simulink model "ADP_2LinkRobot_PEFree_ModFree"  (R2018b)
settings: Solver=ode1  StartTime=0.0  StopTime=100  FixedStep=1/1000  RelTol=1e-3  AbsTol=1e-3  EnableMultiTasking=on
PostLoadFcn:
  | f_Simulink_figureplace
InitFcn:
  | ADP_2LinkRobot_PEFree_ModFree_PreSim
values from neighbouring files (symbols this model uses):
  beta = 0.1    [ADP_2LinkRobot_PEFree_ModFree_PreSim.m]
  etaa1 = 5*(projection==0) + 0.1*(projection==1)    [ADP_2LinkRobot_PEFree_ModFree_PreSim.m]
  etaa2 = 0.001*(projection==0)    [ADP_2LinkRobot_PEFree_ModFree_PreSim.m]
  etac1 = 0.5*(projection==0) + 1*(projection==1)    [ADP_2LinkRobot_PEFree_ModFree_PreSim.m]
  etac2 = 10*(projection==0) + 20*(projection==1)    [ADP_2LinkRobot_PEFree_ModFree_PreSim.m]
  F = 9    [ADP_2LinkRobot_PEFree_ModFree_PreSim.m]
  fs = 1000    [ADP_2LinkRobot_PEFree_ModFree_PreSim.m]
  Gamma0 = 100*eye(L)    [ADP_2LinkRobot_PEFree_ModFree_PreSim.m]
  GammaBar = 100000    [ADP_2LinkRobot_PEFree_ModFree_PreSim.m]
  GammaTheta = diag([95 20 170 20])*(projection==0)+     diag([90 40 160 40])*(projection==1)    [ADP_2LinkRobot_PEFree_ModFree_PreSim.m]
  GG = [GG;phi_pc*Gc*(R\Gc')*phi_pc']    [ADP_2LinkRobot_PEFree_ModFree_PreSim.m]
  k = 10    [ADP_2LinkRobot_PEFree_ModFree_PreSim.m]
  kTheta = 1.1*(projection==0) + 1.1*(projection==1)    [ADP_2LinkRobot_PEFree_ModFree_PreSim.m]
  learning = 1    [ADP_2LinkRobot_PEFree_ModFree_PreSim.m]
  M = 20    [ADP_2LinkRobot_PEFree_ModFree_PreSim.m]
  model = 0    [ADP_2LinkRobot_PEFree_ModFree_PreSim.m]
  N = length(Xc)^4    [ADP_2LinkRobot_PEFree_ModFree_PreSim.m]
  pecutoff = 0.4    [ADP_2LinkRobot_PEFree_ModFree_PreSim.m]
  PHIPF1 = zeros(L,N)    [ADP_2LinkRobot_PEFree_ModFree_PreSim.m]
  PHIPY = [PHIPY;phi_pc*Yc]    [ADP_2LinkRobot_PEFree_ModFree_PreSim.m]
  projection = 1    [ADP_2LinkRobot_PEFree_ModFree_PreSim.m]
  Q = [10 0 0 0; 0 10 0 0; 0 0 1 0; 0 0 0 1]    [ADP_2LinkRobot_PEFree_ModFree_PreSim.m]
  R = 1    [ADP_2LinkRobot_PEFree_ModFree_PreSim.m]
  theta0 = 1*[1; 1; 1; 1]    [ADP_2LinkRobot_PEFree_ModFree_PreSim.m]
  typ = 1    [ADP_2LinkRobot_PEFree_ModFree_PreSim.m]
  v = 0.005    [ADP_2LinkRobot_PEFree_ModFree_PreSim.m]
  WaH0 = 1*WcH0    [ADP_2LinkRobot_PEFree_ModFree_PreSim.m]
  WcH0 = [24.6297684659567,1.18840698913485,2.23807515028947,2.63543366699068,1.16589636116696,0.925620360472737,44.2298481912473,11.2724861339746,3.80631458802382,0.112951648575195]    [ADP_2LinkRobot_PEFree_ModFree_PreSim.m]
  x0 = [1;1;0;0]    [ADP_2LinkRobot_PEFree_ModFree_PreSim.m]
  XQX = zeros(N,1)    [ADP_2LinkRobot_PEFree_ModFree_PreSim.m]
undefined symbols (not defined in the file or in its folder): g
settings Model: Creator=rkamalapurkar  LastModifiedBy=rushik
settings SolverCC: AutoScaleAbsTol=off
settings DataIOCC: LimitDataPoints=on  SaveFormat=Array  SignalLoggingSaveFormat=ModelDataLogs
settings OptimizationCC: ExpressionDepthLimit=2147483647  LifeSpan=inf
settings DebuggingCC: UnderspecifiedInitializationDetection=Classic  MergeDetectMultiDrivingBlocksExec=none  SolverPrmCheckMsg=warning  FcnCallInpInsideContextMsg=warning  StateNameClashWarn=warning  SFUnexpectedBacktrackingDiag=warning  SFNoUnconditionalDefaultTransitionDiag=warning  SFExecutionAtInitializationDiag=none
settings HardwareCC: ProdBitPerPointer=32  ProdBitPerSizeT=32  ProdBitPerPtrDiffT=32  ProdLargestAtomicFloat=None  ProdIntDivRoundTo=Undefined  ProdEndianess=Unspecified  ProdWordSize=32  ProdHWDeviceType=32-bit Generic
settings ModelReferenceCC: PropagateSignalLabelsOutOfModel=off
settings SFSimCC: SimUseLocalCustomCode=off
settings RTWCC: RTWUseLocalCustomCode=off
settings CodeAppCC: StateflowObjectComments=on
settings GRTTargetCC: TargetLangStandard=C89/C90 (ANSI)  GeneratePreprocessorConditionals=Disable all  CombineOutputUpdateFcns=off  GRTInterface=on
settings ConfigComp: CovMetricSettings=dw  CovHtmlReporting=on  CovSaveCumulativeToWorkspaceVar=on  CovSaveSingleToWorkspaceVar=on  CovExternalEMLEnable=off  CovSFcnEnable=off

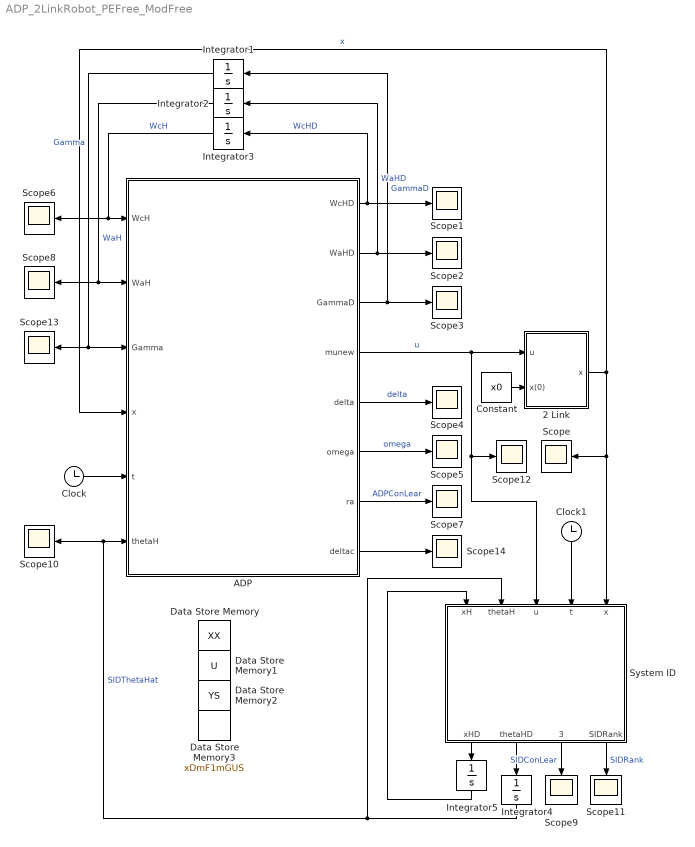
== system ADP_2LinkRobot_PEFree_ModFree ==
  2 Link : Subsystem
  ADP : MATLAB Function  TreatAsAtomicUnit=on
  Clock : Clock
  Clock1 : Clock
  Constant : Constant  Value=x0
  Data Store Memory : DataStoreMemory  DataStoreName=XX  InitialValue=zeros(4,F)  ShowAdditionalParam=off  OutDataTypeStr=double
  Data Store Memory1 : DataStoreMemory  DataStoreName=U  InitialValue=zeros(2,(F+1)/2)  ShowAdditionalParam=off  OutDataTypeStr=double
  Data Store Memory2 : DataStoreMemory  DataStoreName=YS  InitialValue=zeros(4,4*M)  ShowAdditionalParam=off  OutDataTypeStr=double
  Data Store Memory3 : DataStoreMemory  DataStoreName=xDmF1mGUS  InitialValue=zeros(4,M)  ShowAdditionalParam=off  OutDataTypeStr=double
  Integrator1 : Integrator  InitialCondition=Gamma0
  Integrator2 : Integrator  InitialCondition=WaH0
  Integrator3 : Integrator  InitialCondition=WcH0
  Integrator4 : Integrator  InitialCondition=theta0
  Integrator5 : Integrator  InitialCondition=[0;0;0;0]
  Scope{,1..14} (15 alike) : Scope
  System ID : MATLAB Function  TreatAsAtomicUnit=on
  wires:
  ADP/3(GammaD) -> Integrator1/1, Scope3/1  "GammaD"
  ADP/1(WcHD) -> Integrator3/1, Scope1/1  "WcHD"
  Integrator3/1 -> Scope6/1, ADP/1(WcH)  "WcH"
  ADP/2(WaHD) -> Integrator2/1, Scope2/1  "WaHD"
  Integrator2/1 -> ADP/2(WaH), Scope8/1  "WaH"
  ADP/5(delta) -> Scope4/1  "delta"
  ADP/6(omega) -> Scope5/1  "omega"
  Integrator1/1 -> Scope13/1, ADP/3(Gamma)  "Gamma"
  Clock/1 -> ADP/5(t)
  ADP/4(munew) -> System ID/3(u), Scope12/1, 2 Link/1(u)  "u"
  ADP/7(ra) -> Scope7/1  "ADPConLear"
  Integrator4/1 -> System ID/2(thetaH), Scope10/1, ADP/6(thetaH)  "SIDThetaHat"
  2 Link/1(x) -> ADP/4(x), System ID/5(x), Scope/1  "x"
  Constant/1 -> 2 Link/2(x(0))
  System ID/1(xHD) -> Integrator5/1
  Integrator5/1 -> System ID/1(xH)
  System ID/4(SIDRank) -> Scope11/1  "SIDRank"
  System ID/3(SIDConLear) -> Scope9/1  "SIDConLear"
  System ID/2(thetaHD) -> Integrator4/1
  Clock1/1 -> System ID/4(t)
  ADP/8(deltac) -> Scope14/1

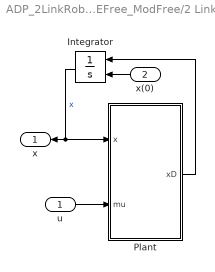
== system ADP_2LinkRobot_PEFree_ModFree/2 Link ==
  u : Inport
  x(0) : Inport  Port=2
  Integrator : Integrator  InitialConditionSource=external  InitialCondition=[1;1;0.0;0.0]
  Plant : MATLAB Function  TreatAsAtomicUnit=on
  x : Outport
  wires:
  Plant/1(xD) -> Integrator/1
  Integrator/1 -> Plant/1(x), x/1  "x"
  u/1 -> Plant/2(mu)
  x(0)/1 -> Integrator/2

== matlab function ADP_2LinkRobot_PEFree_ModFree/2 Link/Plant ==
  data: xD output; x input; mu input
function xD = dynamics(x,mu)
%#codegen

p1=3.473;
p2=.196;
p3=.242;
fd1=5.3;
fd2=1.1;
fs1=8.45;
fs2=2.35;
Minv = (1/(p2^2 - p1*p2 + p3^2*cos(x(2))^2))*...
       [-p2               p2+p3*cos(x(2))  ;...
         p2+p3*cos(x(2)) -p1-2*p3*cos(x(2))];
Vm = [ -p3*sin(x(2))*x(4)  , -p3*sin(x(2))*(x(3)+x(4));
        p3*sin(x(2))*x(3)  , 0                 ];
Fd = diag([fd1,fd2]);
Fs = [fs1*tanh(x(3));fs2*tanh(x(4))];
F = [x(3); x(4); Minv*((-Vm - Fd)*[x(3); x(4)]-Fs)];
G = [0 0; 0 0; Minv];
xD = F+G*mu;

== matlab function ADP_2LinkRobot_PEFree_ModFree/ADP ==
  data: WcH input; WaH input; Gamma input; x input; t input; thetaH input; tf parameter; R parameter; Q parameter; etaa1 parameter; etaa2 parameter; etac1 parameter; v parameter; XQX parameter; GG parameter; PHIPY parameter; PHIPF1 parameter; N parameter; pecutoff parameter; typ parameter; learning parameter; WcHD output; WaHD output; GammaD output; munew output; delta output; omega output size=10,1; ra output; model parameter; etac2 parameter; beta parameter; GammaBar parameter; projection parameter; deltac output
function [WcHD,WaHD,GammaD,munew,delta,omega,ra,deltac]=...
    control(WcH,WaH,Gamma,x,t,thetaH,tf,R,Q,etaa1,etaa2,...
    etac1,v,XQX,GG,PHIPY,PHIPF1,N,pecutoff,typ,learning,model, etac2, beta, GammaBar, projection)
%#codegen
p1=3.473;
p2=.196;
p3=.242;
fd1=5.3;
fd2=1.1;
fs1=8.45;
fs2=2.35;
thetaS=[fd1 fd2 fs1 fs2]';
Minv = (1/(p2^2 - p1*p2 + p3^2*cos(x(2))^2))*...
       [-p2               p2+p3*cos(x(2))  ;...
         p2+p3*cos(x(2)) -p1-2*p3*cos(x(2))];
Vm = [ -p3*sin(x(2))*x(4)  , -p3*sin(x(2))*(x(3)+x(4));
        p3*sin(x(2))*x(3)  , 0                 ];
f1 = [x(3);x(4);-1*Minv*Vm*[x(3);x(4)]];
f2 = [Minv Minv]*diag([x(3);x(4);tanh(1*x(3));tanh(1*x(4))]);
Y = [0 0 0 0;0 0 0 0;-f2];
G = [0 0; 0 0; Minv]; 
% phi = ...
% [x(1)*x(3);...
% x(2)*x(4);...
% x(3)*x(2);...
% x(4)*x(1);...
% x(1)*x(2);...
% x(4)*x(3);...
% x(1)^2;...
% x(3)^2;...
% x(4)^2];
phi_p = ...
[x(3)    0       x(1)    0;...
0       x(4)    0       x(2);...
0       x(3)    x(2)    0;... 
x(4)    0       0       x(1);...
x(2)    x(1)    0       0;...
0       0       x(4)    x(3);...
2*x(1)  0       0       0;...   
0       2*x(2)  0       0;...
0       0       2*x(3)  0;...
0       0       0       2*x(4)];...
mu=-0.5*(R\G')*phi_p'*WaH;
pe = [exp(-0.05*t)*tanh(10*t)*(-10*sin(7*pi*t) + 5*sin(exp(1)*t));...
      exp(-0.05*t)*tanh(10*t)*(-10*sin(9*pi*t) + 10*sin(exp(2)*t))];
% pe = [tanh(10*t)*(-60*sin(7*pi*t) + 10*sin(exp(1)*t));...
%       0];
pe1 = 3*0.85*(tanh(2*t)*(20*sin(sqrt(232)*pi*t)*cos(sqrt(20)*pi*t) + 6*sin(18*exp(2)*t)+ 20*cos(40*t)*cos(21*t)));
pe2 = 0*0.01*(tanh(2*t)*(20*sin(sqrt(132)*pi*t)*cos(sqrt(10)*pi*t) + 6*sin(8*exp(1)*t)+ 20*cos(10*t)*cos(11*t)));
% pe = [pe1;pe2];
munew = mu + pe*(t<=tf*pecutoff)*(learning==2)*(typ==1);
theta = thetaS*(model==1) + thetaH*(model~=1);

%% Concurrent Learning
if typ==1 && learning==1
    GGWaH = reshape(GG*WaH,10,N);
    PHIPYtheta = reshape(PHIPY*theta,10,N);
    deltac = (PHIPF1'+PHIPYtheta')*WcH+XQX-(1/2)*(GGWaH'*WcH)+(1/4)*(GGWaH'*WaH);
    Omegac = (PHIPF1+PHIPYtheta - (1/2)*(GGWaH));
    normm=1./(1.+v.*dot(Omegac.',Omegac.'*Gamma.',2));
    Omegac=Omegac*diag(normm);
    cl = -etac2*Gamma*Omegac*deltac/N;
    ra=real(min(eig(Omegac*diag(normm)*Omegac')));
else
    cl=zeros(10,1);
    GGWaH = 0;
    Omegac = 0;
end

%% ADP
omega = phi_p*(f1+Y*theta+G*mu);
Gsigma = phi_p*G*(R\G')*phi_p';
r = x'*Q*x + mu'*R*mu;
delta = WcH'*omega + r;
rho = (1+v*omega'*(Gamma)*omega);
WcHD = (-etac1*Gamma*omega*delta/rho+cl)*(typ==1);
GammaD = (beta*Gamma-Gamma*(omega*omega'/rho^2)*Gamma)*(typ==1)*(norm(Gamma)<=GammaBar);
WaHD = (etaa1*(WcH-WaH)-etaa2*WaH+etac1*Gsigma'*WaH*omega'*WcH/(4*rho)...
    +etac2*GGWaH*Omegac'*WcH/(4*N))*(typ==1)*(projection==0)...
    +etaa1*(WcH-WaH)*(typ==1)*(projection==1);

== matlab function ADP_2LinkRobot_PEFree_ModFree/System ID ==
  settings: updateMethod=DISCRETE
  data: xH input; xHD output; thetaH input; thetaHD output; u input; SIDConLear output; SIDRank output; t input; x input; k parameter; GammaTheta parameter; kTheta parameter; M parameter; XX data_store_memory; fs parameter; F parameter; g parameter; YS data_store_memory; xDmF1mGUS data_store_memory; U data_store_memory; typ parameter; model parameter
function [xHD,thetaHD,SIDConLear,SIDRank] = Control(xH,thetaH,u,t,x,k,...
                                    GammaTheta,kTheta,M,fs,F,g,typ, model)
%#codegen
% This simulink block implements concurrent-learning based system
% identification using a Savitzky–Golay smoothing filter for state
% derivative computation. 
% fs: Sampling frequency
% M: number of stored data points
% F: Savitzky–Golay filter window length
% g: Savitzky–Golay filter differentiation matrix

global XX; % Data store memory for storing the values of x (initialize 0)
global U; % Data store memory for storing the values of u (initialize 0)
global YS; % Data store memory for storing the values of Y, 
           % made of Y' matrices stacked in a row (initialize 0)
global xDmF1mGUS; % Data store memory for storing the values
                  % of xDot-f1-G*u (initialize 0)

if typ == 1 && model~=1
ite=round(t*fs)+1; % Current iteration number
xT = x-xH;

%Dynamics
p1 = 3.473;
p2 = .196;
p3 = .242;
Minv = (1/(p2^2 - p1*p2 + p3^2*cos(x(2))^2))*...
       [-p2               p2+p3*cos(x(2))  ;...
         p2+p3*cos(x(2)) -p1-2*p3*cos(x(2))];
Vm = [-p3*sin(x(2))*x(4) -p3*sin(x(2))*(x(3)+x(4));
       p3*sin(x(2))*x(3)  0                      ];
f1 = [x(3);x(4);-1*Minv*Vm*[x(3);x(4)]];
f2 = [Minv Minv]*diag([x(3);x(4);tanh(1*x(3));tanh(1*x(4))]);
G = [0 0; 0 0; Minv]; 
Y = [0 0 0 0;0 0 0 0;-f2];

% At every time n store the past F values of the state. Note that 
% Q*g(:,2)/(1/fs) gives the state derivative at n-(F-1)/2
if ite<=F
    XX(:,ite)=x;
else
    XX = [XX(:,2:F) x];
end

% At every time n store the past (F+1)/2 values of the control. Actually, 
% we only need the value of u at n-(F-1)/2. However, I could not find a way
% to store just that single value. Also, even if U is initialized as a row
% vector, MATLAB seems to think its a column.
if ite<=(F+1)/2
    U(:,ite)=u;
else
    U = [U(:,2:(F+1)/2) u];
end

% The state derivative information is only available if ite>=F use
% singular value maximization algorithm to replace elements of YS
% and XDmF1mGUS with new data. At each time ite, the value of the 
% state at ite-(F-1)/2 can be found in XX(:,(F+1)/2)
index=0;
if ite>=F
    xj=XX(:,(F+1)/2);
    Minvj = (1/(p2^2 - p1*p2 + p3^2*cos(xj(2))^2))*...
    [-p2               p2+p3*cos(xj(2))  ;...
    p2+p3*cos(xj(2)) -p1-2*p3*cos(xj(2))];
    f2j = [Minvj Minvj]*diag([xj(3);xj(4);tanh(1*xj(3));tanh(1*xj(4))]);
    Yj = [0 0 0 0;0 0 0 0;-f2j];
    REGste1 = YS*YS';
    svd1=min(svd(REGste1));
    for i=1:M
        YSte=YS; % Store existing data in a temporary variable
        YSte(:,4*i-3:4*i)=Yj'; % Replac i'th Y' matrix with Yj'
        REGste2 = YSte*YSte';
        svd2=min(svd(REGste2)); % Minimum singular value after replacement
        if svd1<svd2 % If replacement results in a higher singular value,
            index=i; % note the index of replacement and
            svd1=svd2; % keep searching for an even higher singular value.           
        end
    end
    
% At this point, index points to the matrix Y' in the stack YS which, when
% replaced with the new matrix Yj', results in the highest singular value.
% If index=0, the new data point is discarded. Otherwise, the stack YS, and
% correspondingly the stack xDmGUS is updated with the new data point. Note
% that since there is a delay of (F-1)/2 for derivative computation, the
% "new" data point we are talking about is the one that was recorded 
% (F-1)/2 steps ago.
    if index ~= 0
        YS(:,4*index-3:4*index)=Yj';
        uj=U(:,1);
        xDj=XX*g(:,2)/(1/fs);
        Vmj = [-p3*sin(xj(2))*xj(4) -p3*sin(xj(2))*(xj(3)+xj(4));
           p3*sin(xj(2))*xj(3)  0                      ];
        f1j = [xj(3);xj(4);-1*Minvj*Vmj*[xj(3);xj(4)]];
        Gj = [0 0; 0 0; Minvj]; 
        xDmF1mGUS(:,index)=xDj-f1j-Gj*uj;
    end
end

xHD = f1 + Y*thetaH + G*u + k*xT;

% Final computation for the concurrent learning-based component of the
% adaptive update law. The concurrent learning component is zero for the
% first F timesteps.
REGs = YS*YS'*(ite>=F);
SIDRank = min(svd(REGs)); % For plots
REG1s = YS*reshape(xDmF1mGUS(:,1:M),4*(M-1+1),1)*(ite>=F);
SIDConLear = (REG1s-REGs*thetaH)/M;
thetaHD = (0*GammaTheta*Y'*xT + kTheta*GammaTheta*SIDConLear);
else
SIDConLear = zeros(size(thetaH));
SIDRank = 0;
xHD = zeros(size(xH));    
thetaHD = zeros(size(thetaH));
end
